simulink model "Vehicle_definitivo_validazione_2"  (R2025b)
settings: Solver=ode4  StartTime=0.0  StopTime=30  FixedStep=0.001  RelTol=1e-3
undefined symbols (not defined in the file): car, new_lotus_bump, new_lotus_roll, new_lotus_steer, posRef, rad, s, Tau_1, Tau_2, Tau_3, Tau_4, yawRef
libraries: aerolibconvert2 x28, simulink_extras x16, simulink x12, slpidlib x2, mpclib x1
(part 2 of 13)

== system Vehicle_definitivo_validazione_2/Driver in the Loop/Vehicle/Tyres1 con relaxation ==
  forces & kinematics : Inport
  T_motor : Inport  Port=2
  T_brake : Inport  Port=3
  J : Inport  Port=4
  Vehicle : Inport  Port=5
  Bus Creator : BusCreator  Inputs=2
  Bus Selector : BusSelector  OutputSignals=Veh_States.velocities.u,Veh_States.velocities.v,Veh_States.velocities.r
  Bus Selector1 : BusSelector  OutputSignals=kinematics.toe,kinematics.camber,kinematics.tyre_deflection,forces.Fz
  Constant9 : Constant  Value=car  OutDataTypeStr=Bus: slBus1
  Integrator : Integrator
  Integrator1 : Integrator
  Integrator2 : Integrator  InitialCondition=car.V0/car.R
  MATLAB Function : MATLAB Function  TreatAsAtomicUnit=on
  Terminator : Terminator
  Terminator1 : Terminator
  tyres ellisse Adams1 : MATLAB Function  TreatAsAtomicUnit=on
  omega_wheels : Outport
  Tire_Forces : Outport  Port=2
  wires:
  Bus Selector/1 -> tyres ellisse Adams1/2(u)  "<u>"
  Bus Selector/2 -> tyres ellisse Adams1/3(v)  "<v>"
  Bus Selector/3 -> tyres ellisse Adams1/4(r)  "<r>"
  tyres ellisse Adams1/3(Fz) -> MATLAB Function/2(Fz)
  Integrator2/1 -> tyres ellisse Adams1/10(omega), omega_wheels/1
  MATLAB Function/1(omega_dot) -> Integrator2/1
  tyres ellisse Adams1/8(Rl) -> MATLAB Function/7(Rl)
  tyres ellisse Adams1/7(T_brake_eff) -> MATLAB Function/6(T_brake_eff)  "T_brake_eff"
  tyres ellisse Adams1/6(T_roll) -> MATLAB Function/5(T_roll)  "T_roll"
  Integrator1/1 -> Bus Creator/2, tyres ellisse Adams1/12(Fy_dyn)  "Fy"
  Integrator/1 -> tyres ellisse Adams1/11(Fx_dyn), MATLAB Function/1(Fx), Bus Creator/1  "Fx"
  tyres ellisse Adams1/2(Fy_dot) -> Integrator1/1  "Fy_dot"
  tyres ellisse Adams1/1(Fx_dot) -> Integrator/1  "Fx_dot"
  tyres ellisse Adams1/5(SR) -> Terminator1/1  "SR"
  tyres ellisse Adams1/4(SA) -> Terminator/1  "SA"
  Bus Selector1/4 -> tyres ellisse Adams1/8("Fz ")  "<Fz>"
  Bus Selector1/3 -> tyres ellisse Adams1/7(tyre_deflection)  "<tyre_deflection>"
  Bus Selector1/2 -> tyres ellisse Adams1/6(camber)  "<camber>"
  Bus Selector1/1 -> tyres ellisse Adams1/5(toe)  "<toe>"
  forces & kinematics/1 -> Bus Selector1/1
  Vehicle/1 -> Bus Selector/1
  Bus Creator/1 -> Tire_Forces/1  "Tire_Forces"
  T_brake/1 -> tyres ellisse Adams1/9(T_brake)
  J/1 -> MATLAB Function/4(J)
  Constant9/1 -> tyres ellisse Adams1/1(car)
  T_motor/1 -> MATLAB Function/3(T_motor)

== system Vehicle_definitivo_validazione_2/Driver in the Loop/Vehicle/Tyres1 senza relaxation ==
  forces & kinematics : Inport
  T_motor : Inport  Port=2
  T_brake : Inport  Port=3
  J : Inport  Port=4
  Veh_States : Inport  Port=5
  Bus Creator : BusCreator  Inputs=2
  Bus Selector : BusSelector  OutputSignals=Veh_States.velocities.u,Veh_States.velocities.v,Veh_States.velocities.r
  Bus Selector1 : BusSelector  OutputSignals=kinematics.toe,kinematics.camber,kinematics.tyre_deflection,forces.Fz
  Constant9 : Constant  Value=car  OutDataTypeStr=Bus: slBus1
  Integrator1 : Integrator  InitialCondition=car.V0/car.R
  Terminator{,1..3} (4 alike) : Terminator
  tyres ellisse Adams1 : MATLAB Function  TreatAsAtomicUnit=on
  omega_wheels : Outport
  Tire_Forces : Outport  Port=2
  wires:
  T_motor/1 -> tyres ellisse Adams1/9(T_motor)
  Bus Selector/3 -> tyres ellisse Adams1/4(r)  "<r>"
  Constant9/1 -> tyres ellisse Adams1/1(car)
  Integrator1/1 -> tyres ellisse Adams1/12(omega), omega_wheels/1  "omega_wheels"
  J/1 -> tyres ellisse Adams1/11(J)
  T_brake/1 -> tyres ellisse Adams1/10(T_brake)
  Bus Selector/1 -> tyres ellisse Adams1/2(u)  "<u>"
  Bus Selector/2 -> tyres ellisse Adams1/3(v)  "<v>"
  tyres ellisse Adams1/1(Fx) -> Bus Creator/1  "Fx"
  tyres ellisse Adams1/2(Fy) -> Bus Creator/2  "Fy"
  Bus Creator/1 -> Tire_Forces/1  "Tire_Forces"
  Veh_States/1 -> Bus Selector/1
  forces & kinematics/1 -> Bus Selector1/1
  Bus Selector1/1 -> tyres ellisse Adams1/5(toe)  "<toe>"
  Bus Selector1/2 -> tyres ellisse Adams1/6(camber)  "<camber>"
  Bus Selector1/3 -> tyres ellisse Adams1/7(tyre_deflection)  "<tyre_deflection>"
  Bus Selector1/4 -> tyres ellisse Adams1/8(Fz)  "<Fz>"
  tyres ellisse Adams1/3(SA) -> Terminator/1  "SA"
  tyres ellisse Adams1/7(omega_dot) -> Integrator1/1
  tyres ellisse Adams1/4(SR) -> Terminator1/1  "SR_i"
  tyres ellisse Adams1/5(T_roll) -> Terminator2/1  "T_roll"
  tyres ellisse Adams1/6(T_brake_eff) -> Terminator3/1  "T_brake_eff"

== system Vehicle_definitivo_validazione_2/Hardware in the Loop/Vehicle/Brakes ==
  BP_tot : Inport
  Constant : Constant  Value=car.bp_max
  Front Caliper : Subsystem
  Gain : Gain  Gain=car.brakebias
  Gain1 : Gain  Gain=1-car.brakebias
  Mux : Mux
  Product2 : Product
  Proportional Valve : Subsystem
  Rear Caliper : Subsystem
  Brake_torque : Outport
  wires:
  Gain/1 -> Front Caliper/1(P_Front)
  Proportional Valve/1(p_rear_mod) -> Rear Caliper/1(P_rear)
  Gain1/1 -> Proportional Valve/1(P_rear)
  Product2/1 -> Gain1/1, Gain/1
  Rear Caliper/1(T_brake_RR) -> Mux/3  "T_brake_RR"
  Rear Caliper/2(T_brake_RL) -> Mux/4  "T_brake_RL"
  Mux/1 -> Brake_torque/1  "Brake_Torque"
  BP_tot/1 -> Product2/1
  Constant/1 -> Product2/2
  Front Caliper/2(T_brake_FL) -> Mux/2  "T_brake_FL"
  Front Caliper/1(T_brake_FR) -> Mux/1  "T_brake_FR"

== system Vehicle_definitivo_validazione_2/Hardware in the Loop/Vehicle/Chassis ==
  Veh_States : Inport
  <steer> : Inport  Port=2
  gear : Inport  Port=3
  Aeromaps : Subsystem
  Bus Creator : BusCreator  Inputs=3
  Bus Creator1 : BusCreator  Inputs=2
  Bus Creator2 : BusCreator  Inputs=2
  Bus Selector : BusSelector  OutputSignals=Veh_States.accelerations.ax_prev,Veh_States.accelerations.ay_prev,Veh_States.velocities.u
  Constant : Constant  Value=0
  Constant12 : Constant  Value=car  OutDataTypeStr=Bus: slBus1
  Constant5 : Constant  Value=car.J_f
  Damper : Subsystem
  Integrator4 : Integrator  InitialCondition=zeros(14,1)
  MATLAB Function4 : MATLAB Function  TreatAsAtomicUnit=on
  MATLAB Function5 : MATLAB Function  TreatAsAtomicUnit=on
  Memory2 : Memory  InheritSampleTime=on
  Memory3 : Memory  InitialCondition=[car.Cz, car.Cx, car.x_cp]  InheritSampleTime=on
  Memory5 : Memory  InitialCondition=[car.IR_spring_front, car.IR_spring_front, car.IR_spring_rear, car.IR_spring_rear, car.tf, car.tr, car.lf, car.lr, car.h_cog, 0.03, 0.04]  InheritSampleTime=on
  Mux : Mux
  Mux2 : Mux
  Terminator : Terminator
  kinematics : Subsystem
  forces & kinematics : Outport
  J : Outport  Port=2
  wires:
  MATLAB Function5/1(dx) -> Integrator4/1
  gear/1 -> MATLAB Function4/1(gear)
  Constant12/1 -> MATLAB Function4/2(car), MATLAB Function5/9(car)
  Mux2/1 -> J/1
  Integrator4/1 -> MATLAB Function5/1(x)
  Memory3/1 -> MATLAB Function5/8(aero_coeffs)
  Constant5/1 -> Mux2/2, Mux2/1
  Memory2/1 -> MATLAB Function5/7(F_damp_in)
  MATLAB Function5/7(corner_rh) -> Aeromaps/1(Ride_height)
  MATLAB Function5/5(susp_vel_ground) -> Damper/1(susp_vel_ground)
  Memory5/1 -> MATLAB Function5/2(kin)
  MATLAB Function5/6(IR) -> Damper/2(IR)
  MATLAB Function4/1(Jr_tot) -> MATLAB Function5/6(Jr_tot), Mux2/4, Mux2/3
  <steer>/1 -> kinematics/1(Steer_Angle)
  MATLAB Function5/8(tyre_deflection) -> Bus Creator/3  "tyre_deflection"
  MATLAB Function5/2(Fz) -> Bus Creator1/1  "Fz"
  MATLAB Function5/3(Drag) -> Bus Creator1/2  "Drag"
  Bus Creator1/1 -> [Forces]  "forces"
  Bus Creator/1 -> Bus Creator2/2  "kinematics"
  [Forces] -> Bus Creator2/1  "forces"
  Bus Creator2/1 -> forces & kinematics/1  "forces & kinematics"
  kinematics/1(kin_dyn) -> [kin]
  kinematics/2(anti%) -> [anti]
  [kin] -> Memory5/1
  Damper/1(F_damper) -> [F_damper]
  [F_damper] -> Memory2/1
  Aeromaps/1(aero_coeff) -> [aero]
  [aero] -> Memory3/1
  Veh_States/1 -> Bus Selector/1
  kinematics/3(camber) -> Bus Creator/1  "camber"
  kinematics/4(toe) -> Bus Creator/2  "toe"
  Constant/1 -> Mux/4, Mux/3, Mux/2, Mux/1
  Mux/1 -> kinematics/2(Wheel_Travel)
  MATLAB Function5/9(damping) -> Terminator/1
  Bus Selector/3 -> MATLAB Function5/5(u)  "<u>"
  Bus Selector/2 -> MATLAB Function5/4(ay_prev)  "<ay_prev>"
  Bus Selector/1 -> MATLAB Function5/3(ax_prev)  "<ax_prev>"

== system Vehicle_definitivo_validazione_2/Hardware in the Loop/Vehicle/Powertrain ==
  tps_ICE : Inport
  omega_wheels : Inport  Port=2
  vehicle : Inport  Port=3
  tps_EM : Inport  Port=4
  bps : Inport  Port=5
  Electric Motor : Subsystem
  Mux : Mux
  pwt con clutch : Subsystem  Commented=on
  pwt senza clutch : Subsystem
  gear : Outport
  torque : Outport  Port=2
  wires:
  tps_ICE/1 -> pwt con clutch/1(tps_ICE), pwt senza clutch/1(tps_ICE)  "tps"
  omega_wheels/1 -> pwt senza clutch/4(omega_wheels), pwt con clutch/2(omega_wheels), Electric Motor/2(omega wheels)
  tps_EM/1 -> Electric Motor/1(tps_EM)
  pwt senza clutch/3(gear) -> gear/1
  Electric Motor/1(T_FR) -> Mux/1  "T_FR"
  Electric Motor/2(T_FL) -> Mux/2  "T_FL"
  pwt senza clutch/1(T_RR) -> Mux/3  "T_RR"
  pwt senza clutch/2(T_RL) -> Mux/4  "T_RL"
  Mux/1 -> torque/1  "torque"
  vehicle/1 -> pwt senza clutch/2(vehicle_states), pwt con clutch/3(vehicle_states)
  bps/1 -> pwt con clutch/4(bps), pwt senza clutch/3(bps)

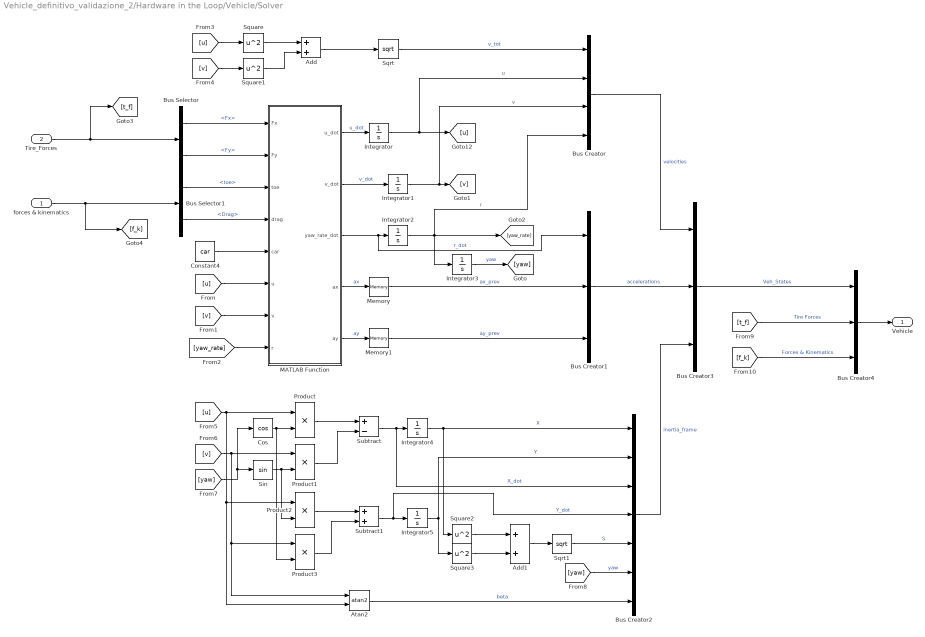
== system Vehicle_definitivo_validazione_2/Hardware in the Loop/Vehicle/Solver ==
  forces & kinematics : Inport
  Tire_Forces : Inport  Port=2
  Add : Sum
  Add1 : Sum
  Atan2 : Trigonometry  Operator=atan2
  Bus Creator : BusCreator  Inputs=4
  Bus Creator1 : BusCreator  Inputs=3
  Bus Creator2 : BusCreator  Inputs=7
  Bus Creator3 : BusCreator  Inputs=3
  Bus Creator4 : BusCreator  Inputs=3
  Bus Selector : BusSelector  OutputSignals=Fx,Fy
  Bus Selector1 : BusSelector  OutputSignals=kinematics.toe,forces.Drag
  Constant4 : Constant  Value=car  OutDataTypeStr=Bus: slBus1
  Cos : Trigonometry  Operator=cos
  Integrator : Integrator  InitialCondition=car.V0
  Integrator{1..5} (5 alike) : Integrator
  MATLAB Function : MATLAB Function  TreatAsAtomicUnit=on
  Memory : Memory
  Memory1 : Memory
  Product{,1..3} (4 alike) : Product
  Sin : Trigonometry
  Sqrt : Sqrt
  Sqrt1 : Sqrt
  Square{,1..3} (4 alike) : Math  Operator=square
  Subtract : Sum  Inputs=+-
  Subtract1 : Sum
  Vehicle : Outport
  wires:
  Subtract/1 -> Bus Creator2/3, Integrator4/1  "X_dot"
  Integrator3/1 -> [yaw]  "yaw"
  [v] -> Atan2/1, Product3/1, Product1/1
  Cos/1 -> Product/2, Product3/2
  MATLAB Function/2(v_dot) -> Integrator1/1  "v_dot"
  Product3/1 -> Subtract1/2
  Integrator5/1 -> Square3/1, Bus Creator2/2  "Y"
  [yaw] -> Cos/1, Sin/1
  Product2/1 -> Subtract1/1
  Integrator4/1 -> Bus Creator2/1, Square2/1  "X"
  MATLAB Function/4(ax) -> Memory/1  "ax"
  [u] -> Product2/1, Atan2/2, Product/1
  [yaw_rate] -> MATLAB Function/8(r)
  Product/1 -> Subtract/1
  Sin/1 -> Product1/2, Product2/2
  Product1/1 -> Subtract/2
  [u] -> MATLAB Function/6(u)
  [v] -> MATLAB Function/7(v)
  MATLAB Function/1(u_dot) -> Integrator/1  "u_dot"
  Subtract1/1 -> Bus Creator2/4, Integrator5/1  "Y_dot"
  MATLAB Function/3(yaw_rate_dot) -> Bus Creator1/1, Integrator2/1  "r_dot"
  Integrator/1 -> [u], Bus Creator/2  "u"
  Memory/1 -> Bus Creator1/2  "ax_prev"
  Memory1/1 -> Bus Creator1/3  "ay_prev"
  Square/1 -> Add/1
  Square1/1 -> Add/2
  Add/1 -> Sqrt/1
  Bus Creator/1 -> Bus Creator3/1  "velocities"
  Bus Creator1/1 -> Bus Creator3/2  "accelerations"
  Bus Creator2/1 -> Bus Creator3/3  "inertia_frame"
  Bus Creator3/1 -> Bus Creator4/1  "Veh_States"
  Constant4/1 -> MATLAB Function/5(car)
  Tire_Forces/1 -> [t_f], Bus Selector/1
  forces & kinematics/1 -> [f_k], Bus Selector1/1
  Bus Selector1/1 -> MATLAB Function/3(toe)  "<toe>"
  Bus Selector1/2 -> MATLAB Function/4(drag)  "<Drag>"
  MATLAB Function/5(ay) -> Memory1/1  "ay"
  Integrator1/1 -> Bus Creator/3, [v]  "v"
  [v] -> Square1/1
  Integrator2/1 -> Bus Creator/4, Integrator3/1, [yaw_rate]  "r"
  Sqrt/1 -> Bus Creator/1  "v_tot"
  [u] -> Square/1
  Square2/1 -> Add1/1
  Square3/1 -> Add1/2
  Add1/1 -> Sqrt1/1
  Sqrt1/1 -> Bus Creator2/5  "S"
  [yaw] -> Bus Creator2/6  "yaw"
  Atan2/1 -> Bus Creator2/7  "beta"
  Bus Selector/2 -> MATLAB Function/2(Fy)  "<Fy>"
  Bus Selector/1 -> MATLAB Function/1(Fx)  "<Fx>"
  [t_f] -> Bus Creator4/2  "Tire Forces"
  [f_k] -> Bus Creator4/3  "Forces & Kinematics"
  Bus Creator4/1 -> Vehicle/1

== system Vehicle_definitivo_validazione_2/Hardware in the Loop/Vehicle/Tyres ==
  forces & kinematics : Inport
  T_motor : Inport  Port=2
  T_brake : Inport  Port=3
  J : Inport  Port=4
  Vehicle : Inport  Port=5
  Bus Creator : BusCreator  Inputs=2
  Bus Selector : BusSelector  OutputSignals=Veh_States.velocities.u,Veh_States.velocities.v,Veh_States.velocities.r
  Bus Selector1 : BusSelector  OutputSignals=kinematics.toe,kinematics.camber,kinematics.tyre_deflection,forces.Fz
  Constant9 : Constant  Value=car  OutDataTypeStr=Bus: slBus1
  Integrator : Integrator
  Integrator1 : Integrator
  Integrator2 : Integrator  InitialCondition=car.V0/car.R
  MATLAB Function : MATLAB Function  TreatAsAtomicUnit=on
  Terminator : Terminator
  Terminator1 : Terminator
  tyres ellisse Adams1 : MATLAB Function  TreatAsAtomicUnit=on
  omega_wheels : Outport
  Tire_Forces : Outport  Port=2
  wires:
  T_motor/1 -> MATLAB Function/3(T_motor)
  Constant9/1 -> tyres ellisse Adams1/1(car)
  J/1 -> MATLAB Function/4(J)
  T_brake/1 -> tyres ellisse Adams1/9(T_brake)
  Bus Creator/1 -> Tire_Forces/1  "Tire_Forces"
  Vehicle/1 -> Bus Selector/1
  forces & kinematics/1 -> Bus Selector1/1
  Bus Selector1/1 -> tyres ellisse Adams1/5(toe)  "<toe>"
  Bus Selector1/2 -> tyres ellisse Adams1/6(camber)  "<camber>"
  Bus Selector1/3 -> tyres ellisse Adams1/7(tyre_deflection)  "<tyre_deflection>"
  Bus Selector1/4 -> tyres ellisse Adams1/8("Fz ")  "<Fz>"
  tyres ellisse Adams1/4(SA) -> Terminator/1  "SA"
  tyres ellisse Adams1/5(SR) -> Terminator1/1  "SR"
  tyres ellisse Adams1/1(Fx_dot) -> Integrator/1  "Fx_dot"
  tyres ellisse Adams1/2(Fy_dot) -> Integrator1/1  "Fy_dot"
  Integrator/1 -> Bus Creator/1, MATLAB Function/1(Fx), tyres ellisse Adams1/11(Fx_dyn)  "Fx"
  Integrator1/1 -> tyres ellisse Adams1/12(Fy_dyn), Bus Creator/2  "Fy"
  tyres ellisse Adams1/6(T_roll) -> MATLAB Function/5(T_roll)  "T_roll"
  tyres ellisse Adams1/7(T_brake_eff) -> MATLAB Function/6(T_brake_eff)  "T_brake_eff"
  tyres ellisse Adams1/8(Rl) -> MATLAB Function/7(Rl)
  MATLAB Function/1(omega_dot) -> Integrator2/1
  Integrator2/1 -> omega_wheels/1, tyres ellisse Adams1/10(omega)
  tyres ellisse Adams1/3(Fz) -> MATLAB Function/2(Fz)
  Bus Selector/3 -> tyres ellisse Adams1/4(r)  "<r>"
  Bus Selector/2 -> tyres ellisse Adams1/3(v)  "<v>"
  Bus Selector/1 -> tyres ellisse Adams1/2(u)  "<u>"

== system Vehicle_definitivo_validazione_2/Senza relaxation/Vehicle/Brakes ==
  BP_tot : Inport
  Constant : Constant  Value=car.bp_max
  Front Caliper : Subsystem
  Gain : Gain  Gain=car.brakebias
  Gain1 : Gain  Gain=1-car.brakebias
  Mux : Mux
  Product2 : Product
  Proportional Valve : Subsystem
  Rear Caliper : Subsystem
  Brake_torque : Outport
  wires:
  Gain/1 -> Front Caliper/1(P_Front)
  Proportional Valve/1(p_rear_mod) -> Rear Caliper/1(P_rear)
  Gain1/1 -> Proportional Valve/1(P_rear)
  Product2/1 -> Gain1/1, Gain/1
  Rear Caliper/1(T_brake_RR) -> Mux/3  "T_brake_RR"
  Rear Caliper/2(T_brake_RL) -> Mux/4  "T_brake_RL"
  Mux/1 -> Brake_torque/1  "Brake_Torque"
  BP_tot/1 -> Product2/1
  Constant/1 -> Product2/2
  Front Caliper/2(T_brake_FL) -> Mux/2  "T_brake_FL"
  Front Caliper/1(T_brake_FR) -> Mux/1  "T_brake_FR"

== system Vehicle_definitivo_validazione_2/Senza relaxation/Vehicle/Chassis ==
  Veh_States : Inport
  <steer> : Inport  Port=2
  gear : Inport  Port=3
  Aeromaps : Subsystem
  Bus Creator : BusCreator  Inputs=3
  Bus Creator1 : BusCreator  Inputs=2
  Bus Creator2 : BusCreator  Inputs=2
  Bus Selector : BusSelector  OutputSignals=Veh_States.accelerations.ax_prev,Veh_States.accelerations.ay_prev,Veh_States.velocities.u
  Constant : Constant  Value=0
  Constant12 : Constant  Value=car  OutDataTypeStr=Bus: slBus1
  Constant5 : Constant  Value=car.J_f
  Damper : Subsystem
  Integrator4 : Integrator  InitialCondition=zeros(14,1)
  MATLAB Function4 : MATLAB Function  TreatAsAtomicUnit=on
  MATLAB Function5 : MATLAB Function  TreatAsAtomicUnit=on
  Memory2 : Memory  InheritSampleTime=on
  Memory3 : Memory  InitialCondition=[car.Cz, car.Cx, car.x_cp]  InheritSampleTime=on
  Memory5 : Memory  InitialCondition=[car.IR_spring_front, car.IR_spring_front, car.IR_spring_rear, car.IR_spring_rear, car.tf, car.tr, car.lf, car.lr, car.h_cog, 0.03, 0.04]  InheritSampleTime=on
  Mux : Mux
  Mux2 : Mux
  Terminator : Terminator
  kinematics : Subsystem
  forces & kinematics : Outport
  J : Outport  Port=2
  wires:
  MATLAB Function5/1(dx) -> Integrator4/1
  gear/1 -> MATLAB Function4/1(gear)
  Constant12/1 -> MATLAB Function4/2(car), MATLAB Function5/9(car)
  Mux2/1 -> J/1
  Integrator4/1 -> MATLAB Function5/1(x)
  Memory3/1 -> MATLAB Function5/8(aero_coeffs)
  Constant5/1 -> Mux2/2, Mux2/1
  Memory2/1 -> MATLAB Function5/7(F_damp_in)
  MATLAB Function5/7(corner_rh) -> Aeromaps/1(Ride_height)
  MATLAB Function5/5(susp_vel_ground) -> Damper/1(susp_vel_ground)
  Memory5/1 -> MATLAB Function5/2(kin)
  MATLAB Function5/6(IR) -> Damper/2(IR)
  MATLAB Function4/1(Jr_tot) -> MATLAB Function5/6(Jr_tot), Mux2/4, Mux2/3
  <steer>/1 -> kinematics/1(Steer_Angle)
  MATLAB Function5/8(tyre_deflection) -> Bus Creator/3  "tyre_deflection"
  MATLAB Function5/2(Fz) -> Bus Creator1/1  "Fz"
  MATLAB Function5/3(Drag) -> Bus Creator1/2  "Drag"
  Bus Creator1/1 -> [Forces]  "forces"
  Bus Creator/1 -> Bus Creator2/2  "kinematics"
  [Forces] -> Bus Creator2/1  "forces"
  Bus Creator2/1 -> forces & kinematics/1  "forces & kinematics"
  kinematics/1(kin_dyn) -> [kin]
  kinematics/2(anti%) -> [anti]
  [kin] -> Memory5/1
  Damper/1(F_damper) -> [F_damper]
  [F_damper] -> Memory2/1
  Aeromaps/1(aero_coeff) -> [aero]
  [aero] -> Memory3/1
  Veh_States/1 -> Bus Selector/1
  kinematics/3(camber) -> Bus Creator/1  "camber"
  kinematics/4(toe) -> Bus Creator/2  "toe"
  Constant/1 -> Mux/4, Mux/3, Mux/2, Mux/1
  Mux/1 -> kinematics/2(Wheel_Travel)
  MATLAB Function5/9(damping) -> Terminator/1
  Bus Selector/3 -> MATLAB Function5/5(u)  "<u>"
  Bus Selector/2 -> MATLAB Function5/4(ay_prev)  "<ay_prev>"
  Bus Selector/1 -> MATLAB Function5/3(ax_prev)  "<ax_prev>"

== system Vehicle_definitivo_validazione_2/Senza relaxation/Vehicle/Powertrain ==
  tps_ICE : Inport
  omega_wheels : Inport  Port=2
  vehicle : Inport  Port=3
  tps_EM : Inport  Port=4
  bps : Inport  Port=5
  Electric Motor : Subsystem
  Mux : Mux
  pwt con clutch : Subsystem  Commented=on
  pwt senza clutch : Subsystem
  gear : Outport
  torque : Outport  Port=2
  wires:
  tps_ICE/1 -> pwt con clutch/1(tps_ICE), pwt senza clutch/1(tps_ICE)  "tps"
  omega_wheels/1 -> pwt senza clutch/4(omega_wheels), pwt con clutch/2(omega_wheels), Electric Motor/2(omega wheels)
  tps_EM/1 -> Electric Motor/1(tps_EM)
  pwt senza clutch/3(gear) -> gear/1
  Electric Motor/1(T_FR) -> Mux/1  "T_FR"
  Electric Motor/2(T_FL) -> Mux/2  "T_FL"
  pwt senza clutch/1(T_RR) -> Mux/3  "T_RR"
  pwt senza clutch/2(T_RL) -> Mux/4  "T_RL"
  Mux/1 -> torque/1  "torque"
  vehicle/1 -> pwt senza clutch/2(vehicle_states), pwt con clutch/3(vehicle_states)
  bps/1 -> pwt con clutch/4(bps), pwt senza clutch/3(bps)

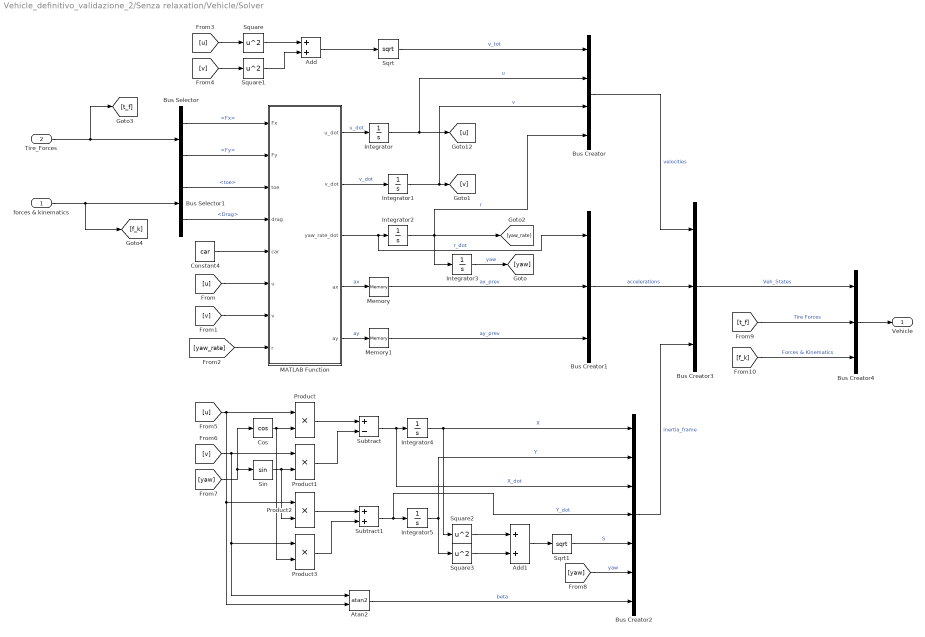
== system Vehicle_definitivo_validazione_2/Senza relaxation/Vehicle/Solver ==
  forces & kinematics : Inport
  Tire_Forces : Inport  Port=2
  Add : Sum
  Add1 : Sum
  Atan2 : Trigonometry  Operator=atan2
  Bus Creator : BusCreator  Inputs=4
  Bus Creator1 : BusCreator  Inputs=3
  Bus Creator2 : BusCreator  Inputs=7
  Bus Creator3 : BusCreator  Inputs=3
  Bus Creator4 : BusCreator  Inputs=3
  Bus Selector : BusSelector  OutputSignals=Fx,Fy
  Bus Selector1 : BusSelector  OutputSignals=kinematics.toe,forces.Drag
  Constant4 : Constant  Value=car  OutDataTypeStr=Bus: slBus1
  Cos : Trigonometry  Operator=cos
  Integrator : Integrator  InitialCondition=car.V0
  Integrator{1..5} (5 alike) : Integrator
  MATLAB Function : MATLAB Function  TreatAsAtomicUnit=on
  Memory : Memory
  Memory1 : Memory
  Product{,1..3} (4 alike) : Product
  Sin : Trigonometry
  Sqrt : Sqrt
  Sqrt1 : Sqrt
  Square{,1..3} (4 alike) : Math  Operator=square
  Subtract : Sum  Inputs=+-
  Subtract1 : Sum
  Vehicle : Outport
  wires:
  Subtract/1 -> Bus Creator2/3, Integrator4/1  "X_dot"
  Integrator3/1 -> [yaw]  "yaw"
  [v] -> Atan2/1, Product3/1, Product1/1
  Cos/1 -> Product/2, Product3/2
  MATLAB Function/2(v_dot) -> Integrator1/1  "v_dot"
  Product3/1 -> Subtract1/2
  Integrator5/1 -> Square3/1, Bus Creator2/2  "Y"
  [yaw] -> Cos/1, Sin/1
  Product2/1 -> Subtract1/1
  Integrator4/1 -> Bus Creator2/1, Square2/1  "X"
  MATLAB Function/4(ax) -> Memory/1  "ax"
  [u] -> Product2/1, Atan2/2, Product/1
  [yaw_rate] -> MATLAB Function/8(r)
  Product/1 -> Subtract/1
  Sin/1 -> Product1/2, Product2/2
  Product1/1 -> Subtract/2
  [u] -> MATLAB Function/6(u)
  [v] -> MATLAB Function/7(v)
  MATLAB Function/1(u_dot) -> Integrator/1  "u_dot"
  Subtract1/1 -> Bus Creator2/4, Integrator5/1  "Y_dot"
  MATLAB Function/3(yaw_rate_dot) -> Bus Creator1/1, Integrator2/1  "r_dot"
  Integrator/1 -> [u], Bus Creator/2  "u"
  Memory/1 -> Bus Creator1/2  "ax_prev"
  Memory1/1 -> Bus Creator1/3  "ay_prev"
  Square/1 -> Add/1
  Square1/1 -> Add/2
  Add/1 -> Sqrt/1
  Bus Creator/1 -> Bus Creator3/1  "velocities"
  Bus Creator1/1 -> Bus Creator3/2  "accelerations"
  Bus Creator2/1 -> Bus Creator3/3  "inertia_frame"
  Bus Creator3/1 -> Bus Creator4/1  "Veh_States"
  Constant4/1 -> MATLAB Function/5(car)
  Tire_Forces/1 -> [t_f], Bus Selector/1
  forces & kinematics/1 -> [f_k], Bus Selector1/1
  Bus Selector1/1 -> MATLAB Function/3(toe)  "<toe>"
  Bus Selector1/2 -> MATLAB Function/4(drag)  "<Drag>"
  MATLAB Function/5(ay) -> Memory1/1  "ay"
  Integrator1/1 -> Bus Creator/3, [v]  "v"
  [v] -> Square1/1
  Integrator2/1 -> Bus Creator/4, Integrator3/1, [yaw_rate]  "r"
  Sqrt/1 -> Bus Creator/1  "v_tot"
  [u] -> Square/1
  Square2/1 -> Add1/1
  Square3/1 -> Add1/2
  Add1/1 -> Sqrt1/1
  Sqrt1/1 -> Bus Creator2/5  "S"
  [yaw] -> Bus Creator2/6  "yaw"
  Atan2/1 -> Bus Creator2/7  "beta"
  Bus Selector/2 -> MATLAB Function/2(Fy)  "<Fy>"
  Bus Selector/1 -> MATLAB Function/1(Fx)  "<Fx>"
  [t_f] -> Bus Creator4/2  "Tire Forces"
  [f_k] -> Bus Creator4/3  "Forces & Kinematics"
  Bus Creator4/1 -> Vehicle/1

== system Vehicle_definitivo_validazione_2/Senza relaxation/Vehicle/Tyres ==
  forces & kinematics : Inport
  T_motor : Inport  Port=2
  T_brake : Inport  Port=3
  J : Inport  Port=4
  Veh_States : Inport  Port=5
  Bus Creator : BusCreator  Inputs=2
  Bus Selector : BusSelector  OutputSignals=Veh_States.velocities.u,Veh_States.velocities.v,Veh_States.velocities.r
  Bus Selector1 : BusSelector  OutputSignals=kinematics.toe,kinematics.camber,kinematics.tyre_deflection,forces.Fz
  Constant9 : Constant  Value=car  OutDataTypeStr=Bus: slBus1
  Integrator1 : Integrator  InitialCondition=car.V0/car.R
  Terminator{,1..3} (4 alike) : Terminator
  tyres ellisse Adams1 : MATLAB Function  TreatAsAtomicUnit=on
  omega_wheels : Outport
  Tire_Forces : Outport  Port=2
  wires:
  T_motor/1 -> tyres ellisse Adams1/9(T_motor)
  Bus Selector/3 -> tyres ellisse Adams1/4(r)  "<r>"
  Constant9/1 -> tyres ellisse Adams1/1(car)
  Integrator1/1 -> tyres ellisse Adams1/12(omega), omega_wheels/1  "omega_wheels"
  J/1 -> tyres ellisse Adams1/11(J)
  T_brake/1 -> tyres ellisse Adams1/10(T_brake)
  Bus Selector/1 -> tyres ellisse Adams1/2(u)  "<u>"
  Bus Selector/2 -> tyres ellisse Adams1/3(v)  "<v>"
  tyres ellisse Adams1/1(Fx) -> Bus Creator/1  "Fx"
  tyres ellisse Adams1/2(Fy) -> Bus Creator/2  "Fy"
  Bus Creator/1 -> Tire_Forces/1  "Tire_Forces"
  Veh_States/1 -> Bus Selector/1
  forces & kinematics/1 -> Bus Selector1/1
  Bus Selector1/1 -> tyres ellisse Adams1/5(toe)  "<toe>"
  Bus Selector1/2 -> tyres ellisse Adams1/6(camber)  "<camber>"
  Bus Selector1/3 -> tyres ellisse Adams1/7(tyre_deflection)  "<tyre_deflection>"
  Bus Selector1/4 -> tyres ellisse Adams1/8(Fz)  "<Fz>"
  tyres ellisse Adams1/3(SA) -> Terminator/1  "SA"
  tyres ellisse Adams1/7(omega_dot) -> Integrator1/1
  tyres ellisse Adams1/4(SR) -> Terminator1/1  "SR_i"
  tyres ellisse Adams1/5(T_roll) -> Terminator2/1  "T_roll"
  tyres ellisse Adams1/6(T_brake_eff) -> Terminator3/1  "T_brake_eff"

== system Vehicle_definitivo_validazione_2/Torque Vectoring/Vehicle/Brakes ==
  BP_tot : Inport
  Constant : Constant  Value=car.bp_max
  Front Caliper : Subsystem
  Gain : Gain  Gain=car.brakebias
  Gain1 : Gain  Gain=1-car.brakebias
  Mux : Mux
  Product2 : Product
  Proportional Valve : Subsystem
  Rear Caliper : Subsystem
  Brake_torque : Outport
  wires:
  Gain/1 -> Front Caliper/1(P_Front)
  Proportional Valve/1(p_rear_mod) -> Rear Caliper/1(P_rear)
  Gain1/1 -> Proportional Valve/1(P_rear)
  Product2/1 -> Gain1/1, Gain/1
  Rear Caliper/1(T_brake_RR) -> Mux/3  "T_brake_RR"
  Rear Caliper/2(T_brake_RL) -> Mux/4  "T_brake_RL"
  Mux/1 -> Brake_torque/1  "Brake_Torque"
  BP_tot/1 -> Product2/1
  Constant/1 -> Product2/2
  Front Caliper/2(T_brake_FL) -> Mux/2  "T_brake_FL"
  Front Caliper/1(T_brake_FR) -> Mux/1  "T_brake_FR"

== system Vehicle_definitivo_validazione_2/Torque Vectoring/Vehicle/Chassis ==
  Veh_States : Inport
  <steer> : Inport  Port=2
  gear : Inport  Port=3
  Aeromaps : Subsystem
  Bus Creator : BusCreator  Inputs=3
  Bus Creator1 : BusCreator  Inputs=2
  Bus Creator2 : BusCreator  Inputs=2
  Bus Selector : BusSelector  OutputSignals=Veh_States.accelerations.ax_prev,Veh_States.accelerations.ay_prev,Veh_States.velocities.u
  Constant : Constant  Value=0
  Constant12 : Constant  Value=car  OutDataTypeStr=Bus: slBus1
  Constant5 : Constant  Value=car.J_f
  Damper : Subsystem
  Integrator4 : Integrator  InitialCondition=zeros(14,1)
  MATLAB Function4 : MATLAB Function  TreatAsAtomicUnit=on
  MATLAB Function5 : MATLAB Function  TreatAsAtomicUnit=on
  Memory2 : Memory  InheritSampleTime=on
  Memory3 : Memory  InitialCondition=[car.Cz, car.Cx, car.x_cp]  InheritSampleTime=on
  Memory5 : Memory  InitialCondition=[car.IR_spring_front, car.IR_spring_front, car.IR_spring_rear, car.IR_spring_rear, car.tf, car.tr, car.lf, car.lr, car.h_cog, 0.03, 0.04]  InheritSampleTime=on
  Mux : Mux
  Mux2 : Mux
  Terminator : Terminator
  kinematics : Subsystem
  forces & kinematics : Outport
  J : Outport  Port=2
  wires:
  MATLAB Function5/1(dx) -> Integrator4/1
  gear/1 -> MATLAB Function4/1(gear)
  Constant12/1 -> MATLAB Function4/2(car), MATLAB Function5/9(car)
  Mux2/1 -> J/1
  Integrator4/1 -> MATLAB Function5/1(x)
  Memory3/1 -> MATLAB Function5/8(aero_coeffs)
  Constant5/1 -> Mux2/2, Mux2/1
  Memory2/1 -> MATLAB Function5/7(F_damp_in)
  MATLAB Function5/7(corner_rh) -> Aeromaps/1(Ride_height)
  MATLAB Function5/5(susp_vel_ground) -> Damper/1(susp_vel_ground)
  Memory5/1 -> MATLAB Function5/2(kin)
  MATLAB Function5/6(IR) -> Damper/2(IR)
  MATLAB Function4/1(Jr_tot) -> MATLAB Function5/6(Jr_tot), Mux2/4, Mux2/3
  <steer>/1 -> kinematics/1(Steer_Angle)
  MATLAB Function5/8(tyre_deflection) -> Bus Creator/3  "tyre_deflection"
  MATLAB Function5/2(Fz) -> Bus Creator1/1  "Fz"
  MATLAB Function5/3(Drag) -> Bus Creator1/2  "Drag"
  Bus Creator1/1 -> [Forces]  "forces"
  Bus Creator/1 -> Bus Creator2/2  "kinematics"
  [Forces] -> Bus Creator2/1  "forces"
  Bus Creator2/1 -> forces & kinematics/1  "forces & kinematics"
  kinematics/1(kin_dyn) -> [kin]
  kinematics/2(anti%) -> [anti]
  [kin] -> Memory5/1
  Damper/1(F_damper) -> [F_damper]
  [F_damper] -> Memory2/1
  Aeromaps/1(aero_coeff) -> [aero]
  [aero] -> Memory3/1
  Veh_States/1 -> Bus Selector/1
  kinematics/3(camber) -> Bus Creator/1  "camber"
  kinematics/4(toe) -> Bus Creator/2  "toe"
  Constant/1 -> Mux/4, Mux/3, Mux/2, Mux/1
  Mux/1 -> kinematics/2(Wheel_Travel)
  MATLAB Function5/9(damping) -> Terminator/1
  Bus Selector/3 -> MATLAB Function5/5(u)  "<u>"
  Bus Selector/2 -> MATLAB Function5/4(ay_prev)  "<ay_prev>"
  Bus Selector/1 -> MATLAB Function5/3(ax_prev)  "<ax_prev>"

== system Vehicle_definitivo_validazione_2/Torque Vectoring/Vehicle/Powertrain ==
  tps_ICE : Inport
  omega_wheels : Inport  Port=2
  vehicle : Inport  Port=3
  T_target : Inport  Port=4
  bps : Inport  Port=5
  Electric Motor : Subsystem
  Mux : Mux
  pwt con clutch : Subsystem  Commented=on
  pwt senza clutch : Subsystem
  gear : Outport
  torque : Outport  Port=2
  wires:
  tps_ICE/1 -> pwt senza clutch/1(tps_ICE), pwt con clutch/1(tps_ICE)  "tps"
  omega_wheels/1 -> pwt con clutch/2(omega_wheels), pwt senza clutch/4(omega_wheels), Electric Motor/2(omega wheels)
  T_target/1 -> Electric Motor/1(T_target)
  pwt senza clutch/3(gear) -> gear/1
  pwt senza clutch/1(T_RR) -> Mux/3  "T_RR"
  pwt senza clutch/2(T_RL) -> Mux/4  "T_RL"
  Mux/1 -> torque/1  "torque"
  vehicle/1 -> pwt senza clutch/2(vehicle_states), pwt con clutch/3(vehicle_states)
  bps/1 -> pwt senza clutch/3(bps), pwt con clutch/4(bps)
  Electric Motor/2(T_FL) -> Mux/2
  Electric Motor/1(T_FR) -> Mux/1

== system Vehicle_definitivo_validazione_2/Torque Vectoring/Vehicle/Powertrain con differenziale1 ==
  tps_ICE : Inport
  omega_wheels : Inport  Port=2
  vehicle states : Inport  Port=3
  Tire_Forces : Inport  Port=4
  tps_EM : Inport  Port=5
  bps : Inport  Port=6
  Electric Motor : Subsystem
  Mux : Mux
  pwt con clutch : Subsystem  Commented=on
  pwt senza clutch : Subsystem
  gear : Outport
  torque : Outport  Port=2
  wires:
  bps/1 -> pwt senza clutch/5(bps), pwt con clutch/5(bps)
  vehicle states/1 -> pwt con clutch/3(vehicle_states), pwt senza clutch/3(vehicle_states)
  Mux/1 -> torque/1  "torque"
  pwt senza clutch/2(T_RL) -> Mux/4  "T_RL"
  pwt senza clutch/1(T_RR) -> Mux/3  "T_RR"
  Electric Motor/2(T_FL) -> Mux/2  "T_FL"
  Electric Motor/1(T_FR) -> Mux/1  "T_FR"
  pwt senza clutch/3(gear) -> gear/1
  tps_EM/1 -> Electric Motor/1(tps_EM)
  Tire_Forces/1 -> pwt senza clutch/4(Tire_Forces), pwt con clutch/4(Tire_Forces)
  omega_wheels/1 -> pwt senza clutch/2(omega_wheels), Electric Motor/2(omega wheels), pwt con clutch/2(omega_wheels)
  tps_ICE/1 -> pwt senza clutch/1(tps_ICE), pwt con clutch/1(tps_ICE)  "tps"

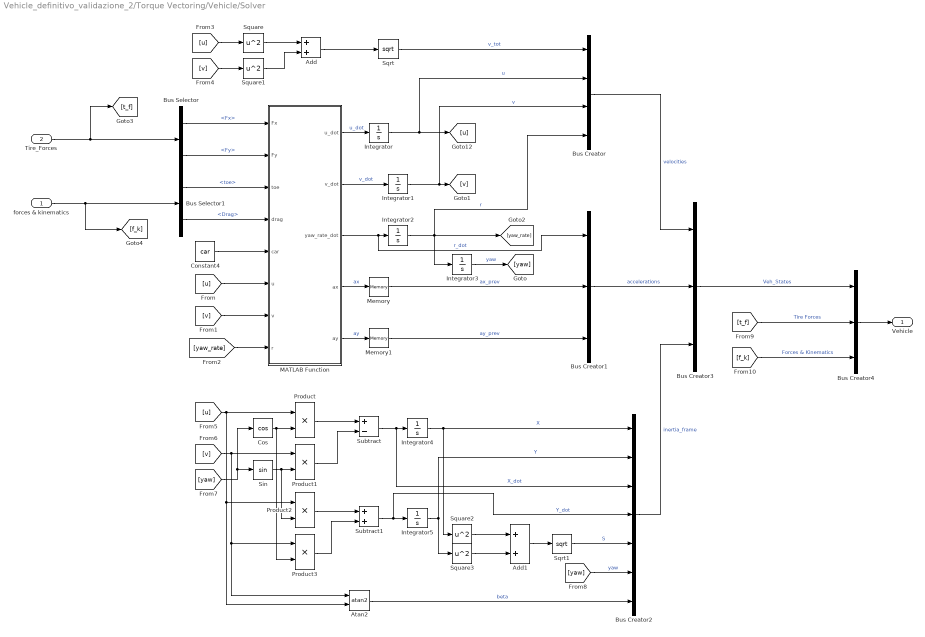
== system Vehicle_definitivo_validazione_2/Torque Vectoring/Vehicle/Solver ==
  forces & kinematics : Inport
  Tire_Forces : Inport  Port=2
  Add : Sum
  Add1 : Sum
  Atan2 : Trigonometry  Operator=atan2
  Bus Creator : BusCreator  Inputs=4
  Bus Creator1 : BusCreator  Inputs=3
  Bus Creator2 : BusCreator  Inputs=7
  Bus Creator3 : BusCreator  Inputs=3
  Bus Creator4 : BusCreator  Inputs=3
  Bus Selector : BusSelector  OutputSignals=Fx,Fy
  Bus Selector1 : BusSelector  OutputSignals=kinematics.toe,forces.Drag
  Constant4 : Constant  Value=car  OutDataTypeStr=Bus: slBus1
  Cos : Trigonometry  Operator=cos
  Integrator : Integrator  InitialCondition=car.V0
  Integrator{1..5} (5 alike) : Integrator
  MATLAB Function : MATLAB Function  TreatAsAtomicUnit=on
  Memory : Memory
  Memory1 : Memory
  Product{,1..3} (4 alike) : Product
  Sin : Trigonometry
  Sqrt : Sqrt
  Sqrt1 : Sqrt
  Square{,1..3} (4 alike) : Math  Operator=square
  Subtract : Sum  Inputs=+-
  Subtract1 : Sum
  Vehicle : Outport
  wires:
  Subtract/1 -> Bus Creator2/3, Integrator4/1  "X_dot"
  Integrator3/1 -> [yaw]  "yaw"
  [v] -> Atan2/1, Product3/1, Product1/1
  Cos/1 -> Product/2, Product3/2
  MATLAB Function/2(v_dot) -> Integrator1/1  "v_dot"
  Product3/1 -> Subtract1/2
  Integrator5/1 -> Square3/1, Bus Creator2/2  "Y"
  [yaw] -> Cos/1, Sin/1
  Product2/1 -> Subtract1/1
  Integrator4/1 -> Bus Creator2/1, Square2/1  "X"
  MATLAB Function/4(ax) -> Memory/1  "ax"
  [u] -> Product2/1, Atan2/2, Product/1
  [yaw_rate] -> MATLAB Function/8(r)
  Product/1 -> Subtract/1
  Sin/1 -> Product1/2, Product2/2
  Product1/1 -> Subtract/2
  [u] -> MATLAB Function/6(u)
  [v] -> MATLAB Function/7(v)
  MATLAB Function/1(u_dot) -> Integrator/1  "u_dot"
  Subtract1/1 -> Bus Creator2/4, Integrator5/1  "Y_dot"
  MATLAB Function/3(yaw_rate_dot) -> Bus Creator1/1, Integrator2/1  "r_dot"
  Integrator/1 -> [u], Bus Creator/2  "u"
  Memory/1 -> Bus Creator1/2  "ax_prev"
  Memory1/1 -> Bus Creator1/3  "ay_prev"
  Square/1 -> Add/1
  Square1/1 -> Add/2
  Add/1 -> Sqrt/1
  Bus Creator/1 -> Bus Creator3/1  "velocities"
  Bus Creator1/1 -> Bus Creator3/2  "accelerations"
  Bus Creator2/1 -> Bus Creator3/3  "inertia_frame"
  Bus Creator3/1 -> Bus Creator4/1  "Veh_States"
  Constant4/1 -> MATLAB Function/5(car)
  Tire_Forces/1 -> [t_f], Bus Selector/1
  forces & kinematics/1 -> [f_k], Bus Selector1/1
  Bus Selector1/1 -> MATLAB Function/3(toe)  "<toe>"
  Bus Selector1/2 -> MATLAB Function/4(drag)  "<Drag>"
  MATLAB Function/5(ay) -> Memory1/1  "ay"
  Integrator1/1 -> Bus Creator/3, [v]  "v"
  [v] -> Square1/1
  Integrator2/1 -> Bus Creator/4, Integrator3/1, [yaw_rate]  "r"
  Sqrt/1 -> Bus Creator/1  "v_tot"
  [u] -> Square/1
  Square2/1 -> Add1/1
  Square3/1 -> Add1/2
  Add1/1 -> Sqrt1/1
  Sqrt1/1 -> Bus Creator2/5  "S"
  [yaw] -> Bus Creator2/6  "yaw"
  Atan2/1 -> Bus Creator2/7  "beta"
  Bus Selector/2 -> MATLAB Function/2(Fy)  "<Fy>"
  Bus Selector/1 -> MATLAB Function/1(Fx)  "<Fx>"
  [t_f] -> Bus Creator4/2  "Tire Forces"
  [f_k] -> Bus Creator4/3  "Forces & Kinematics"
  Bus Creator4/1 -> Vehicle/1

== system Vehicle_definitivo_validazione_2/Torque Vectoring/Vehicle/Tyres ==
  forces & kinematics : Inport
  T_motor : Inport  Port=2
  T_brake : Inport  Port=3
  J : Inport  Port=4
  Vehicle : Inport  Port=5
  Bus Creator : BusCreator  Inputs=2
  Bus Selector : BusSelector  OutputSignals=Veh_States.velocities.u,Veh_States.velocities.v,Veh_States.velocities.r
  Bus Selector1 : BusSelector  OutputSignals=kinematics.toe,kinematics.camber,kinematics.tyre_deflection,forces.Fz
  Constant9 : Constant  Value=car  OutDataTypeStr=Bus: slBus1
  Integrator : Integrator
  Integrator1 : Integrator
  Integrator2 : Integrator  InitialCondition=car.V0/car.R
  MATLAB Function : MATLAB Function  TreatAsAtomicUnit=on
  Terminator : Terminator
  Terminator1 : Terminator
  tyres ellisse Adams1 : MATLAB Function  TreatAsAtomicUnit=on
  omega_wheels : Outport
  Tire_Forces : Outport  Port=2
  wires:
  T_motor/1 -> MATLAB Function/3(T_motor)
  Constant9/1 -> tyres ellisse Adams1/1(car)
  J/1 -> MATLAB Function/4(J)
  T_brake/1 -> tyres ellisse Adams1/9(T_brake)
  Bus Creator/1 -> Tire_Forces/1  "Tire_Forces"
  Vehicle/1 -> Bus Selector/1
  forces & kinematics/1 -> Bus Selector1/1
  Bus Selector1/1 -> tyres ellisse Adams1/5(toe)  "<toe>"
  Bus Selector1/2 -> tyres ellisse Adams1/6(camber)  "<camber>"
  Bus Selector1/3 -> tyres ellisse Adams1/7(tyre_deflection)  "<tyre_deflection>"
  Bus Selector1/4 -> tyres ellisse Adams1/8("Fz ")  "<Fz>"
  tyres ellisse Adams1/4(SA) -> Terminator/1  "SA"
  tyres ellisse Adams1/5(SR) -> Terminator1/1  "SR"
  tyres ellisse Adams1/1(Fx_dot) -> Integrator/1  "Fx_dot"
  tyres ellisse Adams1/2(Fy_dot) -> Integrator1/1  "Fy_dot"
  Integrator/1 -> Bus Creator/1, MATLAB Function/1(Fx), tyres ellisse Adams1/11(Fx_dyn)  "Fx"
  Integrator1/1 -> tyres ellisse Adams1/12(Fy_dyn), Bus Creator/2  "Fy"
  tyres ellisse Adams1/6(T_roll) -> MATLAB Function/5(T_roll)  "T_roll"
  tyres ellisse Adams1/7(T_brake_eff) -> MATLAB Function/6(T_brake_eff)  "T_brake_eff"
  tyres ellisse Adams1/8(Rl) -> MATLAB Function/7(Rl)
  MATLAB Function/1(omega_dot) -> Integrator2/1
  Integrator2/1 -> omega_wheels/1, tyres ellisse Adams1/10(omega)
  tyres ellisse Adams1/3(Fz) -> MATLAB Function/2(Fz)
  Bus Selector/3 -> tyres ellisse Adams1/4(r)  "<r>"
  Bus Selector/2 -> tyres ellisse Adams1/3(v)  "<v>"
  Bus Selector/1 -> tyres ellisse Adams1/2(u)  "<u>"

== system Vehicle_definitivo_validazione_2/Torque Vectoring/Vehicle Control Unit/High Level Controller ==
  Vehicle : Inport
  Driver_in : Inport  Port=2
  Add : Sum  Inputs=-+
  Bus Selector : BusSelector  OutputSignals=Veh_States.velocities.r,Veh_States.velocities.u
  Bus Selector1 : BusSelector  OutputSignals=steer
  Constant12 : Constant  Value=car  OutDataTypeStr=Bus: slBus1
  MATLAB Function : MATLAB Function  TreatAsAtomicUnit=on
  PID Controller : slpidlib/PID Controller  Controller=PID  Form=Parallel  TimeDomain=Continuous-time  UseExternalTs=off  SampleTime=-1  IntegratorMethod=Forward Euler  FilterMethod=Forward Euler  ControllerParametersSource=internal  P=500  I=0  UseKiTs=off  D=50  UseExternalDerivativeSource=off  N=100  UseFilter=on  TunerSelectOption=Transfer Function Based (PID Tuner App)  InitialConditionSource=internal  InitialConditionForIntegrator=0  InitialConditionForFilter=0  DifferentiatorICPrevScaledInput=0  ExternalReset=none  TrackingMode=off  Kt=1  LimitOutput=off  SatLimitsSource=internal  UpperSaturationLimit=inf  LowerSaturationLimit=-inf  LinearizeAsGain=on  AntiWindupMode=none  Kb=1  LimitIntegrator=off  UpperIntegratorSaturationLimit=inf  LowerIntegratorSaturationLimit=-inf  POutMin=[]  POutMax=[]  IOutMin=[]  IOutMax=[]  DOutMin=[]  DOutMax=[]  NOutMin=[]  NOutMax=[]  SumOutMin=[]  SumOutMax=[]  SaturationOutMin=[]  SaturationOutMax=[]  PParamMin=[]  PParamMax=[]  IParamMin=[]  IParamMax=[]  DParamMin=[]  DParamMax=[]  NParamMin=[]  NParamMax=[]  KbParamMin=[]  KbParamMax=[]  KtParamMin=[]  KtParamMax=[]  KbOutMin=[]  KbOutMax=[]  KtOutMin=[]  KtOutMax=[]  IntegratorOutMin=[]  IntegratorOutMax=[]  FilterOutMin=[]  FilterOutMax=[]  SumI1OutMin=[]  SumI1OutMax=[]  SumI2OutMin=[]  SumI2OutMax=[]  SumI3OutMin=[]  SumI3OutMax=[]  SumI4OutMin=[]  SumI4OutMax=[]  SumDOutMin=[]  SumDOutMax=[]  DifferentiatorOutMin=[]  DifferentiatorOutMax=[]  FilterDiffOutCoefMin=[]  FilterDiffOutCoefMax=[]  ReciprocalOutMin=[]  ReciprocalOutMax=[]  SumDenOutMin=[]  SumDenOutMax=[]  SumNumOutMin=[]  SumNumOutMax=[]  DivideOutMin=[]  DivideOutMax=[]  UdiffTsProdOutMin=[]  UdiffTsProdOutMax=[]  NTsProdOutMin=[]  NTsProdOutMax=[]  UintegralTsProdOutMin=[]  UintegralTsProdOutMax=[]  UngainTsProdOutMin=[]  UngainTsProdOutMax=[]  ClampingZeroOutDataTypeStr=Inherit: Inherit via back propagation  ClampingZeroOutMin=[]  ClampingZeroOutMax=[]  FilterDenConstantOutDataTypeStr=Inherit: Inherit via back propagation  FilterDenConstantOutMin=[]  FilterDenConstantOutMax=[]  PCopyOutDataTypeStr=Inherit: Inherit via back propagation  PCopyOutMin=[]  PCopyOutMax=[]  NCopyOutDataTypeStr=Inherit: Inherit via back propagation  NCopyOutMin=[]  NCopyOutMax=[]  IntegratorContinuousStateAttributes=''  IntegratorStateMustResolveToSignalObject=off  IntegratorRTWStateStorageClass=Auto  FilterContinuousStateAttributes=''  FilterStateMustResolveToSignalObject=off  FilterRTWStateStorageClass=Auto  ParallelPVariant=InternalParameters  IdealPVariant=Disabled  IVariant=InternalParameters  DVariant=InternalParameters  IntegratorVariant=Continuous  SatVariant=Disabled  AWVariant=Passthrough  PCopyVariant=Disabled  TRVariant=Disabled  FdbkBlocksVariant=Forward  IdealPFdbkVariant=Disabled  SatFdbkVariant=Disabled  DerivativeFilterVariant=ContFilter  NVariant=InternalParameters  NCopyVariant=Disabled  FilterICVariant=InternalICsFilter  IntegratorICVariant=InternalICs  ExternalResetVariant=Disabled  TRSumVariant=Passthrough  SumFdbkVariant=Disabled  SumVariant=Sum_PID  TsampFilterVariant=InternalTs  TsampNgainVariant=Passthrough  TsampIntegralVariant=Disabled_SignalSpec  ExternalSaturationOutDataTypeStr=Inherit: Same as second input  DerivativeSourceVariant=ErrorSignal  PreIntVariant=InternalPreInt
  Mz_delta : Outport
  wires:
  Vehicle/1 -> Bus Selector/1
  Driver_in/1 -> Bus Selector1/1
  Bus Selector1/1 -> MATLAB Function/2(steer_volante)  "<steer>"
  Constant12/1 -> MATLAB Function/3(car)
  MATLAB Function/1(r_target) -> Add/2  "r_target"
  Add/1 -> PID Controller/1
  PID Controller/1 -> Mz_delta/1
  Bus Selector/2 -> MATLAB Function/1(u)  "<u>"
  Bus Selector/1 -> Add/1  "<r>"

== system Vehicle_definitivo_validazione_2/Torque Vectoring/Vehicle Control Unit/Low Level Controller ==
  Vehicle : Inport
  T_front : Inport  Port=2
  Bus Selector : BusSelector  OutputSignals=Tire Forces.Fy,Forces & Kinematics.forces.Fz
  Constant12 : Constant  Value=car  OutDataTypeStr=Bus: slBus1
  MATLAB Function : MATLAB Function  TreatAsAtomicUnit=on
  Mux : Mux  Inputs=2
  T_target : Outport
  wires:
  Vehicle/1 -> Bus Selector/1
  Bus Selector/1 -> MATLAB Function/1(Fy)  "<Fy>"
  Bus Selector/2 -> MATLAB Function/2(Fz)  "<Fz>"
  T_front/1 -> MATLAB Function/3(T_front)
  Constant12/1 -> MATLAB Function/4(car)
  MATLAB Function/2(T_target_FL) -> Mux/2
  Mux/1 -> T_target/1
  MATLAB Function/1(T_target_FR) -> Mux/1

== system Vehicle_definitivo_validazione_2/Torque Vectoring/Vehicle Control Unit/Torque Allocator ==
  Mz_delta : Inport
  Driver_in : Inport  Port=2
  Bus Selector : BusSelector  OutputSignals=tps_ICE,bps
  Constant12 : Constant  Value=car  OutDataTypeStr=Bus: slBus1
  MATLAB Function : MATLAB Function  TreatAsAtomicUnit=on
  Mux : Mux  Inputs=2
  T_front : Outport
  wires:
  Driver_in/1 -> Bus Selector/1
  Mz_delta/1 -> MATLAB Function/1(Mz_delta)
  Bus Selector/1 -> MATLAB Function/2(tps_ICE)  "<tps_ICE>"
  Bus Selector/2 -> MATLAB Function/3(bps)  "<bps>"
  Constant12/1 -> MATLAB Function/4(car)
  Mux/1 -> T_front/1  "T_front"
  MATLAB Function/1(T_req_FR) -> Mux/1  "T_req_FR"
  MATLAB Function/2(T_req_FL) -> Mux/2  "T_req_FL"

== system Vehicle_definitivo_validazione_2/Con relaxation/Vehicle/Brakes/Front Caliper ==
  P_Front : Inport
  Gain : Gain  Gain=4
  Pad Friction : Gain  Gain=car.brakepad_friction_coeff
  Piston area : Gain  Gain=car.area_front_piston
  brake radius : Gain  Gain=car.brake_radius_front
  from bar to Pascal : Gain  Gain=100000
  T_brake_FR : Outport
  T_brake_FL : Outport  Port=2
  wires:
  P_Front/1 -> from bar to Pascal/1
  Pad Friction/1 -> brake radius/1
  brake radius/1 -> T_brake_FR/1, T_brake_FL/1
  from bar to Pascal/1 -> Gain/1
  Piston area/1 -> Pad Friction/1
  Gain/1 -> Piston area/1

== system Vehicle_definitivo_validazione_2/Con relaxation/Vehicle/Brakes/Proportional Valve ==
  P_rear : Inport
  2-D Lookup Table : Lookup_n-D  BreakpointsForDimension1=[0;3.4473799999999999;6.8947599999999998;10.342140000000001;13.78952;17.236899999999999;20.684280000000001;24.13166;27.579039999999999;31.026420000000002;34.473799999999997;37.92118;41.368560000000002;44.815939999999998;48.26332;51.710700000000003;55.158079999999998;58.605460000000001;62.052840000000003;65.500219999999999;68.947599999999994;72.394980000000004;75.842359999999999;79.289739999999995;82.737120000000004]  BreakpointsForDimension2=[1;2;3;4;5;6;7]  Table=[0 0 0 0 0 0 0;3.4473799999999999 3.4473799999999999 3.4473799999999999 3.4473799999999999 3.4473799999999999 3.4473799999999999 3.4473799999999999;6.8947599999999998 6.8947599999999998 6.8947599999999998 6.8947599999999998 6.8947599999999998 6.8947599999999998 6.8947599999999998;10.342140000000001 10.342140000000001 10.342140000000001 10.342140000000001 10.342140000000001 10.342140000000001 10.342140000000001;11.49126667 13.78952 13.78952 13.78952 13.78952 13.78952 13.78952;12.64039333 17.236899999999999 17.236899999999999 17.236899999999999 17.236899999999999 17.236899999999999 17.236899999999999;13.78952 20.684280000000001 20.684280000000001 20.684280000000001 20.684280000000001 20.684280000000001 20.684280000000001;14.938646670000001 21.833406669999999 24.13166 24.13166 24.13166 24.13166 24.13166;16.087773330000001 22.982533329999999 27.579039999999999 27.579039999999999 27.579039999999999 27.579039999999999 27.579039999999999;17.236899999999999 24.13166 31.026420000000002 31.026420000000002 31.026420000000002 31.026420000000002 31.026420000000002;18.38602667 25.280786670000001 34.473799999999997 34.473799999999997 34.473799999999997 34.473799999999997 34.473799999999997;19.53515333 26.429913330000002 35.458765710000002 37.92118 37.92118 37.92118 37.92118;20.684280000000001 27.579039999999999 36.44373143 41.368560000000002 41.368560000000002 41.368560000000002 41.368560000000002;21.833406669999999 28.72816667 37.428697139999997 42.517686670000003 44.815939999999998 44.815939999999998 44.815939999999998;22.982533329999999 29.877293330000001 38.413662860000002 43.666813329999997 48.26332 48.26332 48.26332;24.13166 31.026420000000002 39.39862857 44.815939999999998 51.710700000000003 51.710700000000003 51.710700000000003;25.280786670000001 32.175546670000003 40.383594289999998 45.965066669999999 52.859826669999997 55.158079999999998 55.158079999999998;26.429913330000002 33.324673330000003 41.368560000000002 47.114193329999999 54.008953329999997 58.605460000000001 58.605460000000001;27.579039999999999 34.473799999999997 42.35352571 48.26332 55.158079999999998 62.052840000000003 62.052840000000003;28.72816667 35.622926669999998 43.338491429999998 49.412446670000001 56.307206669999999 63.201966669999997 65.500219999999999;29.877293330000001 36.772053329999999 44.323457140000002 50.561573330000002 57.45633333 64.351093329999998 68.947599999999994;31.026420000000002 37.92118 45.30842286 51.710700000000003 58.605460000000001 65.500219999999999 70.671289999999999;32.175546670000003 39.070306670000001 46.293388569999998 52.859826669999997 59.754586670000002 66.64934667 72.394980000000004;33.324673330000003 40.219433330000001 47.278354290000003 54.008953329999997 60.903713330000002 67.798473329999993 74.118669999999995;34.473799999999997 41.368560000000002 48.26332 55.158079999999998 62.052840000000003 68.947599999999994 75.842359999999999]  InternalRulePriority=Speed  RndMeth=Simplest
      settings: InputPortMap=u0,u1
  Constant : Constant  Value=car.prop_valve_pos
  p_rear_mod : Outport
  wires:
  P_rear/1 -> 2-D Lookup Table/1
  Constant/1 -> 2-D Lookup Table/2
  2-D Lookup Table/1 -> p_rear_mod/1

== system Vehicle_definitivo_validazione_2/Con relaxation/Vehicle/Brakes/Rear Caliper ==
  P_rear : Inport
  Gain : Gain  Gain=2
  Pad Friction : Gain  Gain=car.brakepad_friction_coeff
  Piston area : Gain  Gain=car.area_rear_piston
  brake radius_rear : Gain  Gain=car.brake_radius_rear
  from bar to Pascal : Gain  Gain=100000
  T_brake_RR : Outport
  T_brake_RL : Outport  Port=2
  wires:
  P_rear/1 -> from bar to Pascal/1
  Pad Friction/1 -> brake radius_rear/1
  brake radius_rear/1 -> T_brake_RL/1, T_brake_RR/1
  from bar to Pascal/1 -> Gain/1
  Gain/1 -> Piston area/1
  Piston area/1 -> Pad Friction/1

== system Vehicle_definitivo_validazione_2/Con relaxation/Vehicle/Chassis/Aeromaps ==
  Ride_height : Inport
  Constant : Constant  Value=car.Cx
  Constant1 : Constant  Value=car.Cz
  Constant2 : Constant  Value=car.x_cp
  Demux : Demux
  Mux : Mux  Inputs=3
  aero_coeff : Outport
  wires:
  Constant/1 -> Mux/1
  Constant1/1 -> Mux/2
  Ride_height/1 -> Demux/1
  Mux/1 -> aero_coeff/1
  Constant2/1 -> Mux/3

== system Vehicle_definitivo_validazione_2/Con relaxation/Vehicle/Chassis/Damper ==
  susp_vel_ground : Inport
  IR : Inport  Port=2
  Demux : Demux
  FL : Subsystem
  FR : Subsystem
  Mux : Mux
  Product : Product
  Product1 : Product
  RL : Subsystem
  RR : Subsystem
  F_damper : Outport
  wires:
  IR/1 -> Product1/2, Product/2
  Product/1 -> Demux/1
  Demux/1 -> FR/1(V_FR)
  FR/1(F_FR) -> Mux/1  "F_FR"
  Mux/1 -> Product1/1
  Demux/2 -> FL/1(V_FL)
  FL/1(F_FL) -> Mux/2  "F_FL"
  Demux/3 -> RR/1(V_RR)
  RR/1(F_RR) -> Mux/3  "F_RR"
  Demux/4 -> RL/1(V_RL)
  RL/1(F_RL) -> Mux/4  "F_RL"
  susp_vel_ground/1 -> Product/1
  Product1/1 -> F_damper/1

== system Vehicle_definitivo_validazione_2/Con relaxation/Vehicle/Chassis/kinematics ==
  Steer_Angle : Inport
  Wheel_Travel : Inport  Port=2
  Add{,1..5} (6 alike) : Sum
  Constant : Constant  Value=car.lf
  Constant1 : Constant  Value=car.lr
  Constant2 : Constant  Value=car.h_cog
  Constant3 : Constant  Value=0.03
  Constant4 : Constant  Value=0.04
  Degrees to Radians : simulink_extras/Transformations/Degrees to Radians
  Demux : Demux
  FL : Subsystem
  FR : Subsystem
  Gain{,1..3} (4 alike) : Gain  Gain=0.5
  Gain4 : Gain  Gain=-1
  Mux : Mux  Inputs=11
  Mux1 : Mux
  Mux2 : Mux
  Mux3 : Mux
  RL : Subsystem
  RR : Subsystem
  Subsystem : Subsystem
  Subsystem1 : Subsystem
  Subtract : Sum  Inputs=-+
  Subtract1 : Sum  Inputs=-+
  kin_dyn : Outport
  anti% : Outport  Port=2
  camber : Outport  Port=3
  toe : Outport  Port=4
  wires:
  Demux/1 -> FR/1(Wheel_Travel), Subtract/1, Add/1
  Add/1 -> Gain/1
  Gain/1 -> Subsystem/1(Heave_F)
  Subtract/1 -> Subsystem/2(Roll_F)
  Demux/3 -> Subtract1/1, Add1/1, RR/1(Wheel_Travel)
  Demux/4 -> RL/1(Wheel_Travel), Add1/2, Subtract1/2
  Add1/1 -> Gain1/1
  Steer_Angle/1 -> FR/2(Steer_Angle), Gain4/1
  Demux/2 -> FL/2(Wheel_Travel), Add/2, Subtract/2
  Mux/1 -> kin_dyn/1
  FR/3(IR_FR) -> Mux/1
  FL/3(IR_FL) -> Mux/2
  RR/3(IR_RR) -> Mux/3
  RL/3(IR_RL) -> Mux/4
  Subsystem/2(tf) -> Mux/5
  Subsystem1/2(tr) -> Mux/6
  FR/1(wb_FR) -> Add2/1
  FL/1(wb_FL) -> Add2/2
  Add2/1 -> Gain2/1
  Gain2/1 -> Add3/1
  Constant/1 -> Add3/2
  Add3/1 -> Mux/7
  Constant1/1 -> Add5/2
  Gain3/1 -> Add5/1
  Add4/1 -> Gain3/1
  Add5/1 -> Mux/8
  RR/1(wb_RR) -> Add4/1
  RL/1(wb_RL) -> Add4/2
  Constant2/1 -> Mux/9
  Mux3/1 -> Degrees to Radians/1
  Mux2/1 -> camber/1
  Mux1/1 -> anti%/1
  FR/2(AD_FR) -> Mux1/1
  FL/2(AD_FL) -> Mux1/2
  RR/2(AS_RR) -> Mux1/3
  RL/2(AS_RL) -> Mux1/4
  FR/4(Camber_FR) -> Mux2/1
  FL/4(Camber_FL) -> Mux2/2
  RR/4(Camber_RR) -> Mux2/3
  RL/4(Camber_RL) -> Mux2/4
  FR/5(Toe_FR) -> Mux3/1
  FL/5(Toe_FL) -> Mux3/2
  RR/5(Toe_RR) -> Mux3/3
  RL/5(Toe_RL) -> Mux3/4
  Gain4/1 -> FL/1(Steer_Angle)
  Constant3/1 -> Mux/10
  Constant4/1 -> Mux/11
  Subtract1/1 -> Subsystem1/2(Roll_R)
  Gain1/1 -> Subsystem1/1(Heave_R)
  Degrees to Radians/1 -> toe/1
  Wheel_Travel/1 -> Demux/1
